simulink model "ConstZeroCondition"  (R2017a)
settings: Solver=VariableStepAuto  StartTime=0.0  StopTime=25  MaxStep=0.01  RelTol=1e-3
settings Model: Creator=Кирилл  LastModifiedBy=drone

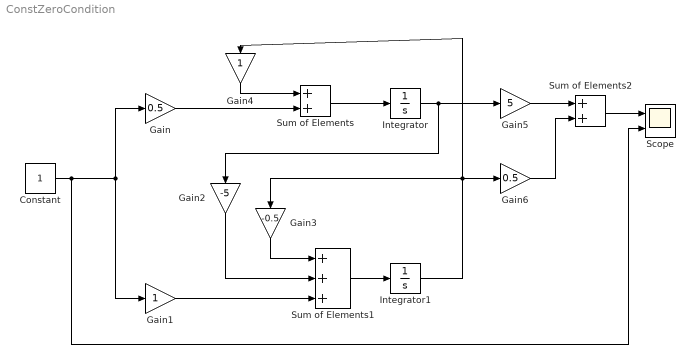
== system ConstZeroCondition ==
  Constant : Constant
  Gain : Gain  Gain=0.5
  Gain1 : Gain
  Gain2 : Gain  Gain=-5
  Gain3 : Gain  Gain=-0.5
  Gain4 : Gain
  Gain5 : Gain  Gain=5
  Gain6 : Gain  Gain=0.5
  Integrator : Integrator
  Integrator1 : Integrator
  Scope : Scope  NumInputPorts=2
  Sum of Elements : Sum  Inputs=2
  Sum of Elements1 : Sum  Inputs=3
  Sum of Elements2 : Sum  Inputs=2
  wires:
  Constant/1 -> Scope/2, Gain/1, Gain1/1
  Gain1/1 -> Sum of Elements1/3
  Sum of Elements/1 -> Integrator/1
  Sum of Elements1/1 -> Integrator1/1
  Integrator/1 -> Gain2/1, Gain5/1
  Integrator1/1 -> Gain6/1, Gain3/1, Gain4/1
  Sum of Elements2/1 -> Scope/1
  Gain5/1 -> Sum of Elements2/1
  Gain6/1 -> Sum of Elements2/2
  Gain2/1 -> Sum of Elements1/2
  Gain3/1 -> Sum of Elements1/1
  Gain4/1 -> Sum of Elements/1
  Gain/1 -> Sum of Elements/2
